simulink model "RemoteController"  (R2014b)
settings: Solver=ode45  StartTime=0.0  StopTime=endtime_selfdefine  RelTol=1e-3
values from neighbouring files (symbols this model uses):
  flight_mode = 1    [flight_control_run.m]
  simple_mode = 2    [flight_control_run.m]
undefined symbols (not defined in the file or in its folder): sigbuilder_block
settings Model: Creator=Ehang  LastModifiedBy=Ehang
settings DebuggingCC: SignalInfNanChecking=error  InheritedTsInSrcMsg=none  UnconnectedInputMsg=none  UnconnectedOutputMsg=none  UnconnectedLineMsg=none
settings ModelReferenceCC: ModelReferenceNumInstancesAllowed=Single

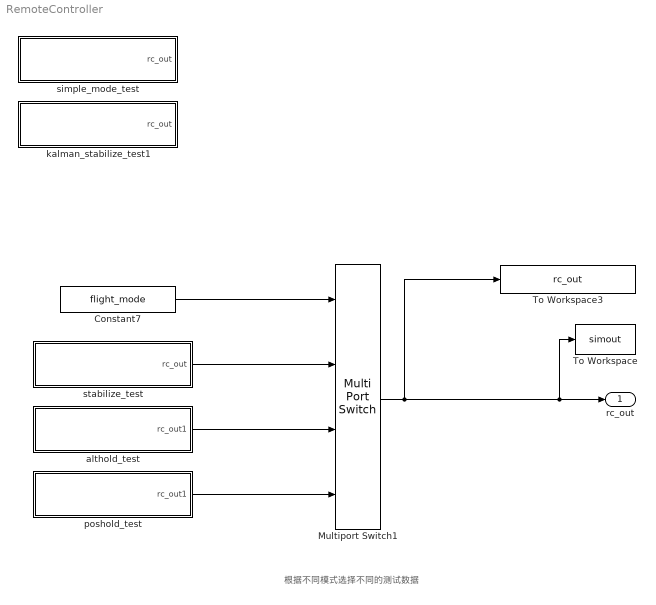
== system RemoteController ==
  note: 根据不同模式选择不同的测试数据
  Constant7 : Constant  Value=flight_mode  SampleTime=0.0025
  Multiport Switch1 : MultiPortSwitch
  To Workspace : ToWorkspace  VariableName=simout  SaveFormat=Structure  SampleTime=-1
  To Workspace3 : ToWorkspace  VariableName=rc_out  SaveFormat=Structure  SampleTime=-1
  althold_test : Subsystem
  kalman_stabilize_test1 : Subsystem
  poshold_test : Subsystem
  simple_mode_test : Subsystem
  stabilize_test : Subsystem
  rc_out : Outport
  wires:
  Multiport Switch1/1 -> To Workspace/1, rc_out/1, To Workspace3/1
  Constant7/1 -> Multiport Switch1/1
  althold_test/1(rc_out1) -> Multiport Switch1/3
  poshold_test/1(rc_out1) -> Multiport Switch1/4
  stabilize_test/1(rc_out) -> Multiport Switch1/2

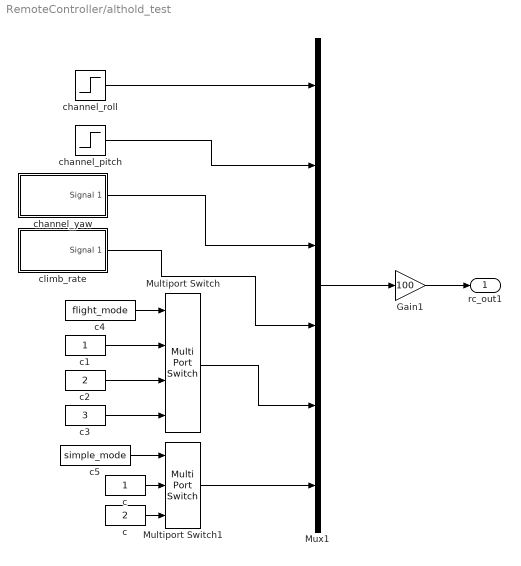
== system RemoteController/althold_test ==
  Gain1 : Gain  Gain=100  SampleTime=0.0025
  Multiport Switch : MultiPortSwitch
  Multiport Switch1 : MultiPortSwitch  Inputs=2
  Mux1 : Mux  Inputs=6
  c : Constant  SampleTime=-1
  "c " : Constant  Value=2  SampleTime=-1
  c1 : Constant  SampleTime=-1
  c2 : Constant  Value=2  SampleTime=-1
  c3 : Constant  Value=3  SampleTime=-1
  c4 : Constant  Value=flight_mode  SampleTime=-1
  c5 : Constant  Value=simple_mode  SampleTime=-1
  channel_pitch : Step  Time=2.5  After=15  SampleTime=0.0025
  channel_roll : Step  Time=2  After=25  SampleTime=0.0025
  channel_yaw : Subsystem  Tag=STV Subsys  LoadFcn=sigbuilder_block('load');  StartFcn=sigbuilder_block('start');  StopFcn=sigbuilder_block('stop');  ClipboardFcn=sigbuilder_block('clipboard');  mask(Sigbuilder block){}
      mask help: Simulink:masks:SigbuilderBlock_MD
      mask init:
      | if ~strcmp(get_param(bdroot(gcbh),'SimulationStatus'),'stopped') tuvar = sigbuilder_block('maskInit'); end
      settings: CopyFcn=sigbuilder_block('copy');  DeleteFcn=sigbuilder_block('delete');  ModelCloseFcn=sigbuilder_block('modelClose');  PreSaveFcn=sigbuilder_block('preSave');  PauseFcn=sigbuilder_block('pause')  ContinueFcn=sigbuilder_block('continue')  NameChangeFcn=sigbuilder_block('namechange');  OpenFcn=sigbuilder_block('open',[437.25 117.75 550.5 393.75 ]);  CloseFcn=sigbuilder_block('close');
      mask Display: plot(0, 0, 100, 100,[2, 2, 32, 32, 2], [68, 8, 8, 68, 68],[32, 2], [38, 38], [32, 19, 2],[53, 60, 44], [32, 17, 17, 2],[16, 16, 31, 31]);txt = getActiveGroup(gcbh);text(2, 100, txt,'verticalAlignment', 'top');
  climb_rate : Subsystem  Tag=STV Subsys  LoadFcn=sigbuilder_block('load');  StartFcn=sigbuilder_block('start');  StopFcn=sigbuilder_block('stop');  ClipboardFcn=sigbuilder_block('clipboard');  mask(Sigbuilder block){}
      mask help: Simulink:masks:SigbuilderBlock_MD
      mask init:
      | if ~strcmp(get_param(bdroot(gcbh),'SimulationStatus'),'stopped') tuvar = sigbuilder_block('maskInit'); end
      settings: CopyFcn=sigbuilder_block('copy');  DeleteFcn=sigbuilder_block('delete');  ModelCloseFcn=sigbuilder_block('modelClose');  PreSaveFcn=sigbuilder_block('preSave');  PauseFcn=sigbuilder_block('pause')  ContinueFcn=sigbuilder_block('continue')  NameChangeFcn=sigbuilder_block('namechange');  OpenFcn=sigbuilder_block('open',[437.25 117.75 550.5 393.75 ]);  CloseFcn=sigbuilder_block('close');
      mask Display: plot(0, 0, 100, 100,[2, 2, 32, 32, 2], [68, 8, 8, 68, 68],[32, 2], [38, 38], [32, 19, 2],[53, 60, 44], [32, 17, 17, 2],[16, 16, 31, 31]);txt = getActiveGroup(gcbh);text(2, 100, txt,'verticalAlignment', 'top');
  rc_out1 : Outport
  wires:
  Mux1/1 -> Gain1/1
  Gain1/1 -> rc_out1/1
  climb_rate/1(Signal 1) -> Mux1/4
  channel_roll/1 -> Mux1/1
  channel_pitch/1 -> Mux1/2
  channel_yaw/1(Signal 1) -> Mux1/3
  Multiport Switch1/1 -> Mux1/6
  c1/1 -> Multiport Switch/2
  c2/1 -> Multiport Switch/3
  c3/1 -> Multiport Switch/4
  Multiport Switch/1 -> Mux1/5
  c4/1 -> Multiport Switch/1
  c5/1 -> Multiport Switch1/1
  c/1 -> Multiport Switch1/2
  "c "/1 -> Multiport Switch1/3

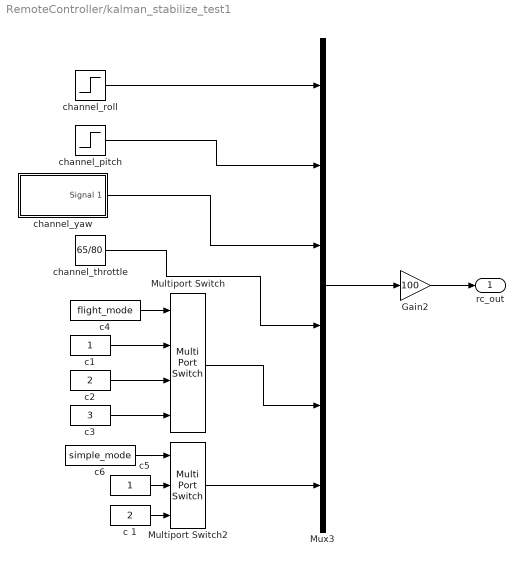
== system RemoteController/kalman_stabilize_test1 ==
  Gain2 : Gain  Gain=100  SampleTime=0.0025
  Multiport Switch : MultiPortSwitch
  Multiport Switch2 : MultiPortSwitch  Inputs=2
  Mux3 : Mux  Inputs=6
  c 1 : Constant  Value=2  SampleTime=-1
  c1 : Constant  SampleTime=-1
  c2 : Constant  Value=2  SampleTime=-1
  c3 : Constant  Value=3  SampleTime=-1
  c4 : Constant  Value=flight_mode  SampleTime=-1
  c5 : Constant  SampleTime=-1
  c6 : Constant  Value=simple_mode  SampleTime=-1
  channel_pitch : Step  Time=2.5  After=35  SampleTime=0.0025
  channel_roll : Step  Time=2  After=25  SampleTime=0.0025
  channel_throttle : Constant  Value=65/80  SampleTime=-1
  channel_yaw : Subsystem  Tag=STV Subsys  LoadFcn=sigbuilder_block('load');  StartFcn=sigbuilder_block('start');  StopFcn=sigbuilder_block('stop');  ClipboardFcn=sigbuilder_block('clipboard');  mask(Sigbuilder block){}
      mask help: Simulink:masks:SigbuilderBlock_MD
      mask init:
      | if ~strcmp(get_param(bdroot(gcbh),'SimulationStatus'),'stopped') tuvar = sigbuilder_block('maskInit'); end
      settings: CopyFcn=sigbuilder_block('copy');  DeleteFcn=sigbuilder_block('delete');  ModelCloseFcn=sigbuilder_block('modelClose');  PreSaveFcn=sigbuilder_block('preSave');  PauseFcn=sigbuilder_block('pause')  ContinueFcn=sigbuilder_block('continue')  NameChangeFcn=sigbuilder_block('namechange');  OpenFcn=sigbuilder_block('open',[437.25 117.75 550.5 393.75 ]);  CloseFcn=sigbuilder_block('close');
      mask Display: plot(0, 0, 100, 100,[2, 2, 32, 32, 2], [68, 8, 8, 68, 68],[32, 2], [38, 38], [32, 19, 2],[53, 60, 44], [32, 17, 17, 2],[16, 16, 31, 31]);txt = getActiveGroup(gcbh);text(2, 100, txt,'verticalAlignment', 'top');
  rc_out : Outport
  wires:
  Mux3/1 -> Gain2/1
  Gain2/1 -> rc_out/1
  channel_throttle/1 -> Mux3/4
  channel_roll/1 -> Mux3/1
  channel_pitch/1 -> Mux3/2
  channel_yaw/1(Signal 1) -> Mux3/3
  c1/1 -> Multiport Switch/2
  c2/1 -> Multiport Switch/3
  c3/1 -> Multiport Switch/4
  Multiport Switch/1 -> Mux3/5
  c4/1 -> Multiport Switch/1
  Multiport Switch2/1 -> Mux3/6
  c6/1 -> Multiport Switch2/1
  c5/1 -> Multiport Switch2/2
  c 1/1 -> Multiport Switch2/3

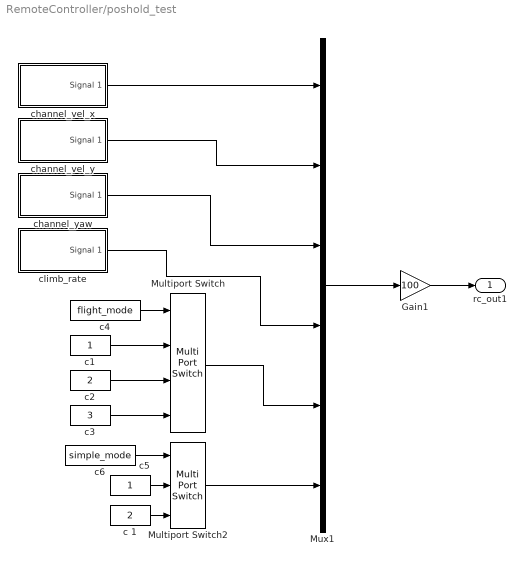
== system RemoteController/poshold_test ==
  Gain1 : Gain  Gain=100  SampleTime=0.0025
  Multiport Switch : MultiPortSwitch
  Multiport Switch2 : MultiPortSwitch  Inputs=2
  Mux1 : Mux  Inputs=6
  c 1 : Constant  Value=2  SampleTime=-1
  c1 : Constant  SampleTime=-1
  c2 : Constant  Value=2  SampleTime=-1
  c3 : Constant  Value=3  SampleTime=-1
  c4 : Constant  Value=flight_mode  SampleTime=-1
  c5 : Constant  SampleTime=-1
  c6 : Constant  Value=simple_mode  SampleTime=-1
  channel_vel_x : Subsystem  Tag=STV Subsys  LoadFcn=sigbuilder_block('load');  StartFcn=sigbuilder_block('start');  StopFcn=sigbuilder_block('stop');  ClipboardFcn=sigbuilder_block('clipboard');  mask(Sigbuilder block){}
      mask help: Simulink:masks:SigbuilderBlock_MD
      mask init:
      | if ~strcmp(get_param(bdroot(gcbh),'SimulationStatus'),'stopped') tuvar = sigbuilder_block('maskInit'); end
      settings: CopyFcn=sigbuilder_block('copy');  DeleteFcn=sigbuilder_block('delete');  ModelCloseFcn=sigbuilder_block('modelClose');  PreSaveFcn=sigbuilder_block('preSave');  PauseFcn=sigbuilder_block('pause')  ContinueFcn=sigbuilder_block('continue')  NameChangeFcn=sigbuilder_block('namechange');  OpenFcn=sigbuilder_block('open',[437.25 117.75 550.5 393.75 ]);  CloseFcn=sigbuilder_block('close');
      mask Display: plot(0, 0, 100, 100,[2, 2, 32, 32, 2], [68, 8, 8, 68, 68],[32, 2], [38, 38], [32, 19, 2],[53, 60, 44], [32, 17, 17, 2],[16, 16, 31, 31]);txt = getActiveGroup(gcbh);text(2, 100, txt,'verticalAlignment', 'top');
  "channel_vel_y " : Subsystem  Tag=STV Subsys  LoadFcn=sigbuilder_block('load');  StartFcn=sigbuilder_block('start');  StopFcn=sigbuilder_block('stop');  ClipboardFcn=sigbuilder_block('clipboard');  mask(Sigbuilder block){}
      mask help: Simulink:masks:SigbuilderBlock_MD
      mask init:
      | if ~strcmp(get_param(bdroot(gcbh),'SimulationStatus'),'stopped') tuvar = sigbuilder_block('maskInit'); end
      settings: CopyFcn=sigbuilder_block('copy');  DeleteFcn=sigbuilder_block('delete');  ModelCloseFcn=sigbuilder_block('modelClose');  PreSaveFcn=sigbuilder_block('preSave');  PauseFcn=sigbuilder_block('pause')  ContinueFcn=sigbuilder_block('continue')  NameChangeFcn=sigbuilder_block('namechange');  OpenFcn=sigbuilder_block('open',[437.25 117.75 550.5 393.75 ]);  CloseFcn=sigbuilder_block('close');
      mask Display: plot(0, 0, 100, 100,[2, 2, 32, 32, 2], [68, 8, 8, 68, 68],[32, 2], [38, 38], [32, 19, 2],[53, 60, 44], [32, 17, 17, 2],[16, 16, 31, 31]);txt = getActiveGroup(gcbh);text(2, 100, txt,'verticalAlignment', 'top');
  channel_yaw : Subsystem  Tag=STV Subsys  LoadFcn=sigbuilder_block('load');  StartFcn=sigbuilder_block('start');  StopFcn=sigbuilder_block('stop');  ClipboardFcn=sigbuilder_block('clipboard');  mask(Sigbuilder block){}
      mask help: Simulink:masks:SigbuilderBlock_MD
      mask init:
      | if ~strcmp(get_param(bdroot(gcbh),'SimulationStatus'),'stopped') tuvar = sigbuilder_block('maskInit'); end
      settings: CopyFcn=sigbuilder_block('copy');  DeleteFcn=sigbuilder_block('delete');  ModelCloseFcn=sigbuilder_block('modelClose');  PreSaveFcn=sigbuilder_block('preSave');  PauseFcn=sigbuilder_block('pause')  ContinueFcn=sigbuilder_block('continue')  NameChangeFcn=sigbuilder_block('namechange');  OpenFcn=sigbuilder_block('open',[437.25 117.75 550.5 393.75 ]);  CloseFcn=sigbuilder_block('close');
      mask Display: plot(0, 0, 100, 100,[2, 2, 32, 32, 2], [68, 8, 8, 68, 68],[32, 2], [38, 38], [32, 19, 2],[53, 60, 44], [32, 17, 17, 2],[16, 16, 31, 31]);txt = getActiveGroup(gcbh);text(2, 100, txt,'verticalAlignment', 'top');
  climb_rate : Subsystem  Tag=STV Subsys  LoadFcn=sigbuilder_block('load');  StartFcn=sigbuilder_block('start');  StopFcn=sigbuilder_block('stop');  ClipboardFcn=sigbuilder_block('clipboard');  mask(Sigbuilder block){}
      mask help: Simulink:masks:SigbuilderBlock_MD
      mask init:
      | if ~strcmp(get_param(bdroot(gcbh),'SimulationStatus'),'stopped') tuvar = sigbuilder_block('maskInit'); end
      settings: CopyFcn=sigbuilder_block('copy');  DeleteFcn=sigbuilder_block('delete');  ModelCloseFcn=sigbuilder_block('modelClose');  PreSaveFcn=sigbuilder_block('preSave');  PauseFcn=sigbuilder_block('pause')  ContinueFcn=sigbuilder_block('continue')  NameChangeFcn=sigbuilder_block('namechange');  OpenFcn=sigbuilder_block('open',[437.25 117.75 550.5 393.75 ]);  CloseFcn=sigbuilder_block('close');
      mask Display: plot(0, 0, 100, 100,[2, 2, 32, 32, 2], [68, 8, 8, 68, 68],[32, 2], [38, 38], [32, 19, 2],[53, 60, 44], [32, 17, 17, 2],[16, 16, 31, 31]);txt = getActiveGroup(gcbh);text(2, 100, txt,'verticalAlignment', 'top');
  rc_out1 : Outport
  wires:
  Mux1/1 -> Gain1/1
  Gain1/1 -> rc_out1/1
  climb_rate/1(Signal 1) -> Mux1/4
  channel_vel_x/1(Signal 1) -> Mux1/1
  "channel_vel_y "/1(Signal 1) -> Mux1/2
  channel_yaw/1(Signal 1) -> Mux1/3
  c1/1 -> Multiport Switch/2
  c2/1 -> Multiport Switch/3
  c3/1 -> Multiport Switch/4
  Multiport Switch/1 -> Mux1/5
  c4/1 -> Multiport Switch/1
  c6/1 -> Multiport Switch2/1
  c5/1 -> Multiport Switch2/2
  c 1/1 -> Multiport Switch2/3
  Multiport Switch2/1 -> Mux1/6

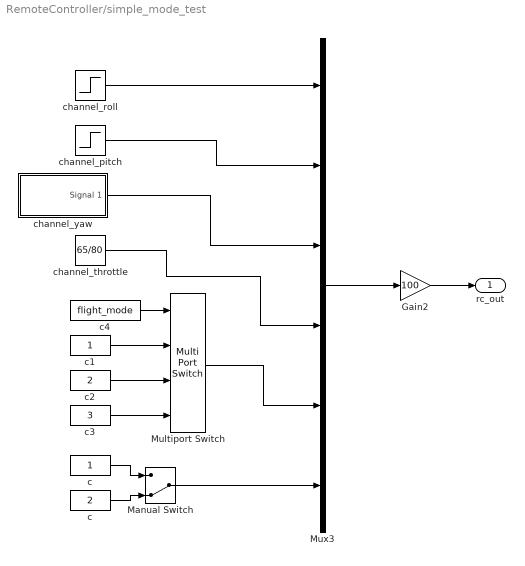
== system RemoteController/simple_mode_test ==
  Gain2 : Gain  Gain=100  SampleTime=0.0025
  Manual Switch : ManualSwitch  CurrentSetting=0
  Multiport Switch : MultiPortSwitch
  Mux3 : Mux  Inputs=6
  c : Constant  SampleTime=-1
  "c " : Constant  Value=2  SampleTime=-1
  c1 : Constant  SampleTime=-1
  c2 : Constant  Value=2  SampleTime=-1
  c3 : Constant  Value=3  SampleTime=-1
  c4 : Constant  Value=flight_mode  SampleTime=-1
  channel_pitch : Step  Time=2.5  After=0  SampleTime=0.0025
  channel_roll : Step  Time=5  After=25  SampleTime=0.0025
  channel_throttle : Constant  Value=65/80  SampleTime=-1
  channel_yaw : Subsystem  Tag=STV Subsys  LoadFcn=sigbuilder_block('load');  StartFcn=sigbuilder_block('start');  StopFcn=sigbuilder_block('stop');  ClipboardFcn=sigbuilder_block('clipboard');  mask(Sigbuilder block){}
      mask help: Simulink:masks:SigbuilderBlock_MD
      mask init:
      | if ~strcmp(get_param(bdroot(gcbh),'SimulationStatus'),'stopped') tuvar = sigbuilder_block('maskInit'); end
      settings: CopyFcn=sigbuilder_block('copy');  DeleteFcn=sigbuilder_block('delete');  ModelCloseFcn=sigbuilder_block('modelClose');  PreSaveFcn=sigbuilder_block('preSave');  PauseFcn=sigbuilder_block('pause')  ContinueFcn=sigbuilder_block('continue')  NameChangeFcn=sigbuilder_block('namechange');  OpenFcn=sigbuilder_block('open',[437.25 117.75 550.5 393.75 ]);  CloseFcn=sigbuilder_block('close');
      mask Display: plot(0, 0, 100, 100,[2, 2, 32, 32, 2], [68, 8, 8, 68, 68],[32, 2], [38, 38], [32, 19, 2],[53, 60, 44], [32, 17, 17, 2],[16, 16, 31, 31]);txt = getActiveGroup(gcbh);text(2, 100, txt,'verticalAlignment', 'top');
  rc_out : Outport
  wires:
  Mux3/1 -> Gain2/1
  Gain2/1 -> rc_out/1
  channel_throttle/1 -> Mux3/4
  channel_roll/1 -> Mux3/1
  channel_pitch/1 -> Mux3/2
  channel_yaw/1(Signal 1) -> Mux3/3
  c/1 -> Manual Switch/1
  "c "/1 -> Manual Switch/2
  Manual Switch/1 -> Mux3/6
  c1/1 -> Multiport Switch/2
  c2/1 -> Multiport Switch/3
  c3/1 -> Multiport Switch/4
  Multiport Switch/1 -> Mux3/5
  c4/1 -> Multiport Switch/1

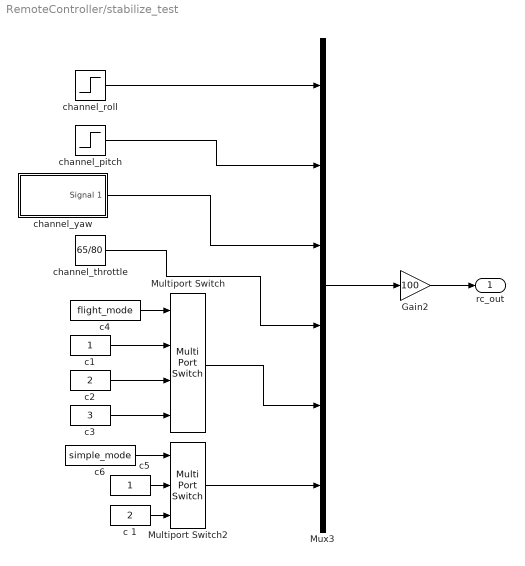
== system RemoteController/stabilize_test ==
  Gain2 : Gain  Gain=100  SampleTime=0.0025
  Multiport Switch : MultiPortSwitch
  Multiport Switch2 : MultiPortSwitch  Inputs=2
  Mux3 : Mux  Inputs=6
  c 1 : Constant  Value=2  SampleTime=-1
  c1 : Constant  SampleTime=-1
  c2 : Constant  Value=2  SampleTime=-1
  c3 : Constant  Value=3  SampleTime=-1
  c4 : Constant  Value=flight_mode  SampleTime=-1
  c5 : Constant  SampleTime=-1
  c6 : Constant  Value=simple_mode  SampleTime=-1
  channel_pitch : Step  Time=2.5  After=15  SampleTime=0.0025
  channel_roll : Step  Time=2  After=-25  SampleTime=0.0025
  channel_throttle : Constant  Value=65/80  SampleTime=-1
  channel_yaw : Subsystem  Tag=STV Subsys  LoadFcn=sigbuilder_block('load');  StartFcn=sigbuilder_block('start');  StopFcn=sigbuilder_block('stop');  ClipboardFcn=sigbuilder_block('clipboard');  mask(Sigbuilder block){}
      mask help: Simulink:masks:SigbuilderBlock_MD
      mask init:
      | if ~strcmp(get_param(bdroot(gcbh),'SimulationStatus'),'stopped') tuvar = sigbuilder_block('maskInit'); end
      settings: CopyFcn=sigbuilder_block('copy');  DeleteFcn=sigbuilder_block('delete');  ModelCloseFcn=sigbuilder_block('modelClose');  PreSaveFcn=sigbuilder_block('preSave');  PauseFcn=sigbuilder_block('pause')  ContinueFcn=sigbuilder_block('continue')  NameChangeFcn=sigbuilder_block('namechange');  OpenFcn=sigbuilder_block('open',[437.25 117.75 550.5 393.75 ]);  CloseFcn=sigbuilder_block('close');
      mask Display: plot(0, 0, 100, 100,[2, 2, 32, 32, 2], [68, 8, 8, 68, 68],[32, 2], [38, 38], [32, 19, 2],[53, 60, 44], [32, 17, 17, 2],[16, 16, 31, 31]);txt = getActiveGroup(gcbh);text(2, 100, txt,'verticalAlignment', 'top');
  rc_out : Outport
  wires:
  Mux3/1 -> Gain2/1
  Gain2/1 -> rc_out/1
  channel_throttle/1 -> Mux3/4
  channel_roll/1 -> Mux3/1
  channel_pitch/1 -> Mux3/2
  channel_yaw/1(Signal 1) -> Mux3/3
  c1/1 -> Multiport Switch/2
  c2/1 -> Multiport Switch/3
  c3/1 -> Multiport Switch/4
  Multiport Switch/1 -> Mux3/5
  c4/1 -> Multiport Switch/1
  Multiport Switch2/1 -> Mux3/6
  c6/1 -> Multiport Switch2/1
  c5/1 -> Multiport Switch2/2
  c 1/1 -> Multiport Switch2/3

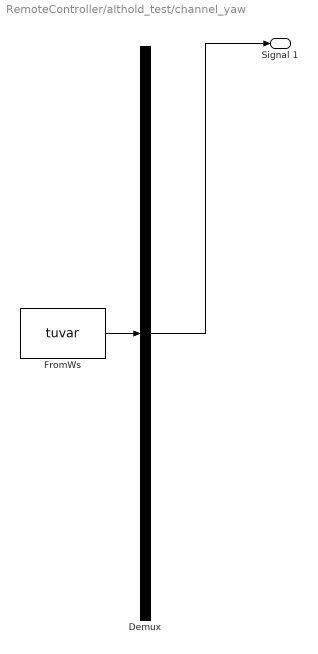
== system RemoteController/althold_test/channel_yaw ==
  Demux : Demux  Tag=STV Demux  Outputs=1
  FromWs : FromWorkspace  Tag=STV FromWs  VariableName=tuvar  SampleTime=0
      SigBuilderData=|
      | common.afterFinalStr = 'Extrapolate'
      | common.sampleTime = 0
      | dataSet.timeRange = [0 10]
      | dataSet.name = 'Group 1'
      | sbobj.Groups.Name = 'Group 1'
      | sbobj.Groups.Signals.Name = 'Signal 1'
      | sbobj.Groups.Signals.XData = [0 6.02 6.02 8 8 10]
      | sbobj.Groups.Signals.YData = [0 0 15 15 0 0]
  Signal 1 : Outport  Tag=STV Outport
  wires:
  Demux/1 -> Signal 1/1
  FromWs/1 -> Demux/1

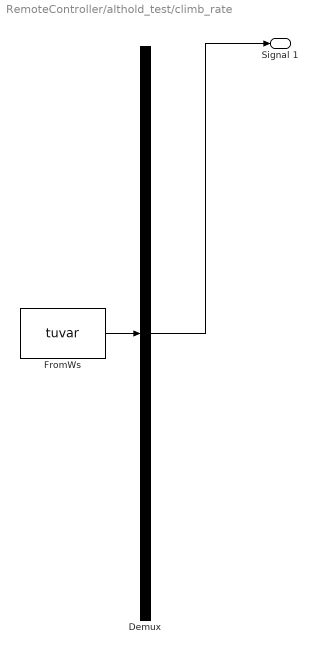
== system RemoteController/althold_test/climb_rate ==
  Demux : Demux  Tag=STV Demux  Outputs=1
  FromWs : FromWorkspace  Tag=STV FromWs  VariableName=tuvar  SampleTime=0
      SigBuilderData=|
      | common.afterFinalStr = 'Extrapolate'
      | common.sampleTime = 0
      | dataSet.timeRange = [0 10]
      | dataSet.name = 'Group 1'
      | sbobj.Groups.Name = 'Group 1'
      | sbobj.Groups.Signals.Name = 'Signal 1'
      | sbobj.Groups.Signals.XData = [0 0.98 0.98 4 4 10]
      | sbobj.Groups.Signals.YData = [0 0 300 300 0 0]
  Signal 1 : Outport  Tag=STV Outport
  wires:
  Demux/1 -> Signal 1/1
  FromWs/1 -> Demux/1

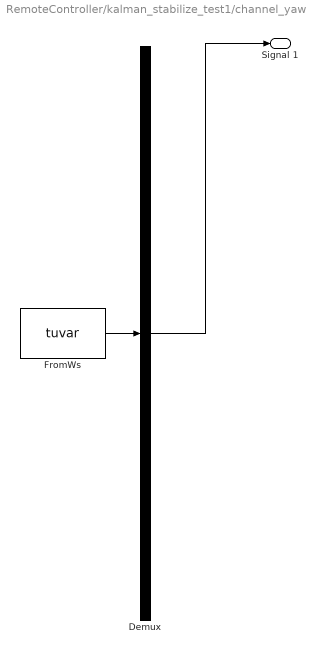
== system RemoteController/kalman_stabilize_test1/channel_yaw ==
  Demux : Demux  Tag=STV Demux  Outputs=1
  FromWs : FromWorkspace  Tag=STV FromWs  VariableName=tuvar  SampleTime=0
      SigBuilderData=|
      | common.afterFinalStr = 'Extrapolate'
      | common.sampleTime = 0
      | dataSet.timeRange = [0 10]
      | dataSet.name = 'Group 1'
      | sbobj.Groups.Name = 'Group 1'
      | sbobj.Groups.Signals.Name = 'Signal 1'
      | sbobj.Groups.Signals.XData = [0 5.98 5.98 7.98 7.98 10]
      | sbobj.Groups.Signals.YData = [0 0 15 15 0 0]
  Signal 1 : Outport  Tag=STV Outport
  wires:
  Demux/1 -> Signal 1/1
  FromWs/1 -> Demux/1

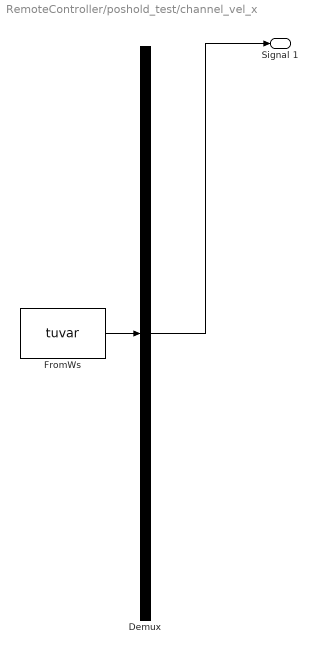
== system RemoteController/poshold_test/channel_vel_x ==
  Demux : Demux  Tag=STV Demux  Outputs=1
  FromWs : FromWorkspace  Tag=STV FromWs  VariableName=tuvar  SampleTime=0
      SigBuilderData=|
      | common.afterFinalStr = 'Extrapolate'
      | common.sampleTime = 0
      | dataSet.timeRange = [0 10]
      | dataSet.name = 'Group 1'
      | sbobj.Groups.Name = 'Group 1'
      | sbobj.Groups.Signals.Name = 'Signal 1'
      | sbobj.Groups.Signals.XData = [0 3.98 3.98 5.98 5.98 10]
      | sbobj.Groups.Signals.YData = [0 0 300 300 0 0]
  Signal 1 : Outport  Tag=STV Outport
  wires:
  Demux/1 -> Signal 1/1
  FromWs/1 -> Demux/1

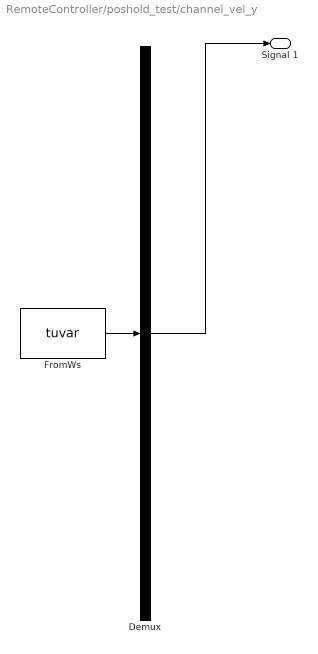
== system RemoteController/poshold_test/channel_vel_y  ==
  Demux : Demux  Tag=STV Demux  Outputs=1
  FromWs : FromWorkspace  Tag=STV FromWs  VariableName=tuvar  SampleTime=0
      SigBuilderData=|
      | common.afterFinalStr = 'Extrapolate'
      | common.sampleTime = 0
      | dataSet.timeRange = [0 10]
      | dataSet.name = 'Group 1'
      | sbobj.Groups.Name = 'Group 1'
      | sbobj.Groups.Signals.Name = 'Signal 1'
      | sbobj.Groups.Signals.XData = [0 7 7 9 9 10]
      | sbobj.Groups.Signals.YData = [0 0 200 200 0 0]
  Signal 1 : Outport  Tag=STV Outport
  wires:
  Demux/1 -> Signal 1/1
  FromWs/1 -> Demux/1

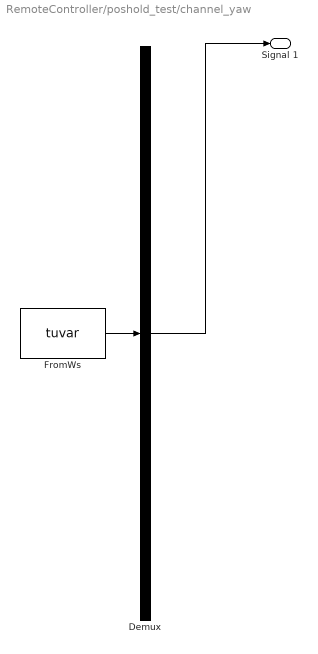
== system RemoteController/poshold_test/channel_yaw ==
  Demux : Demux  Tag=STV Demux  Outputs=1
  FromWs : FromWorkspace  Tag=STV FromWs  VariableName=tuvar  SampleTime=0
      SigBuilderData=|
      | common.afterFinalStr = 'Extrapolate'
      | common.sampleTime = 0
      | dataSet.timeRange = [0 10]
      | dataSet.name = 'Group 1'
      | sbobj.Groups.Name = 'Group 1'
      | sbobj.Groups.Signals.Name = 'Signal 1'
      | sbobj.Groups.Signals.XData = [0 0.98 0.98 3 3 10]
      | sbobj.Groups.Signals.YData = [0 0 15 15 0 0]
  Signal 1 : Outport  Tag=STV Outport
  wires:
  Demux/1 -> Signal 1/1
  FromWs/1 -> Demux/1

== system RemoteController/poshold_test/climb_rate ==
  Demux : Demux  Tag=STV Demux  Outputs=1
  FromWs : FromWorkspace  Tag=STV FromWs  VariableName=tuvar  SampleTime=0
      SigBuilderData=|
      | common.afterFinalStr = 'Extrapolate'
      | common.sampleTime = 0
      | dataSet.timeRange = [0 10]
      | dataSet.name = 'Group 1'
      | sbobj.Groups.Name = 'Group 1'
      | sbobj.Groups.Signals.Name = 'Signal 1'
      | sbobj.Groups.Signals.XData = [0 0.98 0.98 3.98 3.98 10]
      | sbobj.Groups.Signals.YData = [0 0 300 300 0 0]
  Signal 1 : Outport  Tag=STV Outport
  wires:
  Demux/1 -> Signal 1/1
  FromWs/1 -> Demux/1

== system RemoteController/simple_mode_test/channel_yaw ==
  Demux : Demux  Tag=STV Demux  Outputs=1
  FromWs : FromWorkspace  Tag=STV FromWs  VariableName=tuvar  SampleTime=0
      SigBuilderData=|
      | common.afterFinalStr = 'Extrapolate'
      | common.sampleTime = 0
      | dataSet.timeRange = [0 10]
      | dataSet.name = 'Group 1'
      | sbobj.Groups.Name = 'Group 1'
      | sbobj.Groups.Signals.Name = 'Signal 1'
      | sbobj.Groups.Signals.XData = [0 0.98 0.98 3 3 10]
      | sbobj.Groups.Signals.YData = [0 0 15 15 0 0]
  Signal 1 : Outport  Tag=STV Outport
  wires:
  Demux/1 -> Signal 1/1
  FromWs/1 -> Demux/1

== system RemoteController/stabilize_test/channel_yaw ==
  Demux : Demux  Tag=STV Demux  Outputs=1
  FromWs : FromWorkspace  Tag=STV FromWs  VariableName=tuvar  SampleTime=0
      SigBuilderData=|
      | common.afterFinalStr = 'Extrapolate'
      | common.sampleTime = 0
      | dataSet.timeRange = [0 10]
      | dataSet.name = 'Group 1'
      | sbobj.Groups.Name = 'Group 1'
      | sbobj.Groups.Signals.Name = 'Signal 1'
      | sbobj.Groups.Signals.XData = [0 5.98 5.98 7.98 7.98 10]
      | sbobj.Groups.Signals.YData = [0 0 15 15 0 0]
  Signal 1 : Outport  Tag=STV Outport
  wires:
  Demux/1 -> Signal 1/1
  FromWs/1 -> Demux/1
